simulink model "acceleration"  (R2022a)
settings: Solver=VariableStepAuto  StartTime=0.0  StopTime=10  RelTol=1e-3
settings Model: Creator=amani  LastModifiedBy=amani

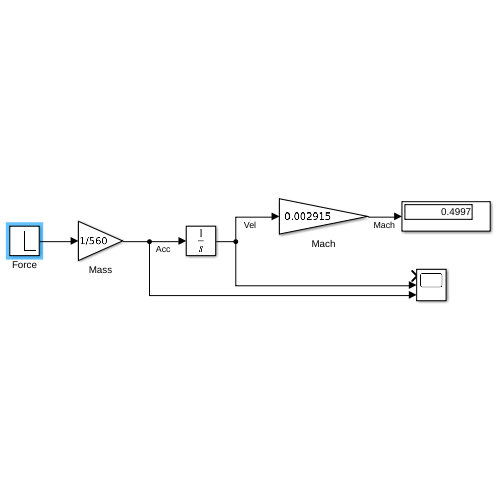
[thumbnail: Simulink's stored preview of the top-level diagram]
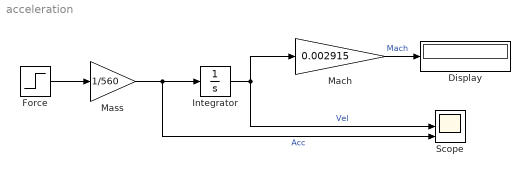
== system acceleration ==
  Display : Display
  Force : Step  Time=3  Before=32000  After=0  SampleTime=0
  Integrator : Integrator
  Mach : Gain  Gain=0.002915
  Mass : Gain  Gain=1/560
  Scope : Scope  NumInputPorts=3
  wires:
  Integrator/1 -> Mach/1, Scope/2  "Vel"
  Force/1 -> Mass/1
  Mass/1 -> Integrator/1, Scope/3  "Acc"
  Mach/1 -> Display/1  "Mach"
